simulink model "A1_VSC_3phase"  (R2024b)
settings: Solver=ode1  StartTime=0.0  StopTime=tsim  FixedStep=tsamp  RelTol=1e-3
values from neighbouring files (symbols this model uses):
  conv = 4    [A1_VSC_3phase.m]
  fsw = 35e3    (= 35000)    [A1_VSC_3phase.m]
  kd = sqrt(2/3)    [A1_VSC_3phase.m]
  Ki = 2*pi*fsw*req/10    (= 659.734457254)    [A1_VSC_3phase.m]
  ko = sqrt(1/3)    [A1_VSC_3phase.m]
  Kp = 2*pi*fsw*Lg/10    (= 43.9822971503)    [A1_VSC_3phase.m]
  Lg = 2e-3    (= 0.002)    [A1_VSC_3phase.m]
  P1 = -5e3    (= -5000)    [A1_VSC_3phase.m]
  P2 = 1e3    (= 1000)    [A1_VSC_3phase.m]
  P3 = 5e3    (= 5000)    [A1_VSC_3phase.m]
  P4 = -5e3    (= -5000)    [A1_VSC_3phase.m]
  rg = 10e-3    (= 0.01)    [A1_VSC_3phase.m]
  tsamp = 1/(samples_per_switching*fsw)    (= 2.85714285714e-07)    [A1_VSC_3phase.m]
  Vdc = 800    [A1_VSC_3phase.m]
  Vg1 = 428    [A1_VSC_3phase.m]
  Vg2 = 438    [A1_VSC_3phase.m]
  Vg3 = 438    [A1_VSC_3phase.m]
  Vg4 = 438    [A1_VSC_3phase.m]
libraries: spsMosfetLib x6, spsVoltageMeasurementLib x4, spsControlledVoltageSourceLib x3, spsCurrentMeasurementLib x3, spsSeriesRLCBranchLib x3, slpidlib x2, spsStairGeneratorLib x2, spsDCVoltageSourceLib x1, simulink x1, spsGroundLib x1, spsPLL3phLib x1, spspowerguiLib x1
settings Model: Creator=Admin  LastModifiedBy=admin
settings RTWCC: GPUComputeCapability=3.5

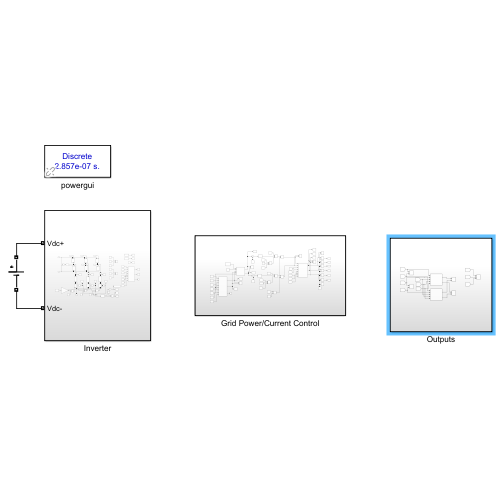
[thumbnail: Simulink's stored preview of the top-level diagram]
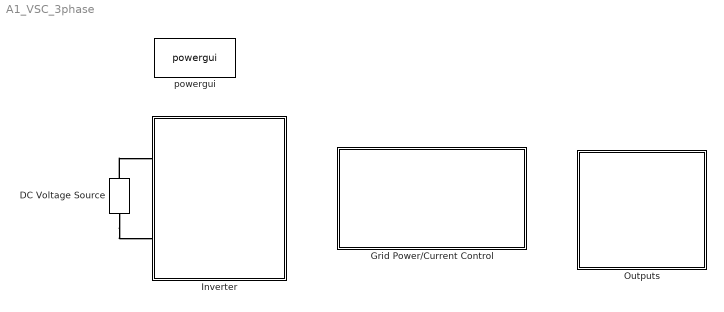
== system A1_VSC_3phase ==
  DC Voltage Source : spsDCVoltageSourceLib/DC Voltage Source  Amplitude=Vdc  Measurements=None
  Grid Power/Current Control : Subsystem
  Inverter : Subsystem
  Outputs : Subsystem
  powergui : spspowerguiLib/powergui  Priority=1  SimulationMode=Discrete  SampleTime=tsamp  frequency=60  Iterations=50  frequencyindice=0  Pbase=100e6  ErrMax=1e-4  UnitsV=kV  UnitsW=MW  buscounter=0  FunctionMessages=off  echomessages=off  EnableUseOfTLC=off  CurrentSourceSwitches=off  DisableSnubberDevices=off  DisableRonSwitches=off  DisableVfSwitches=off  DisplayEquations=off  AutomaticDiscreteSolvers=off  SolverType=Tustin/Backward Euler (TBE)  Interpol=off  ExternalGateDelay=off  methode=off  Ts=100  x0status=blocks  SPID=on  SwTol=0  HookPort=off  NonlinearTolerance=1e-4  nMaxIteration=100  ContinueOnMaxIteration=off  RestoreLinks=warning  ResistiveCurrentMeasurement=off  Frange=[0:2:500]  Ylog=off  Xlog=on  ShowGrid=off  save=off  variable=ZData  structure=0  ZoomFFT=off  StartTime=0.0  cycles=1  DisplayStyle=1  fundamental=60  FreqAxis=off  MaxFrequency=1000  frequencyindicesteady=1  RmsSteady=1  display=off
  connections:
  DC Voltage Source/LConn1 -- Inverter/LConn2
  DC Voltage Source/RConn1 -- Inverter/LConn1

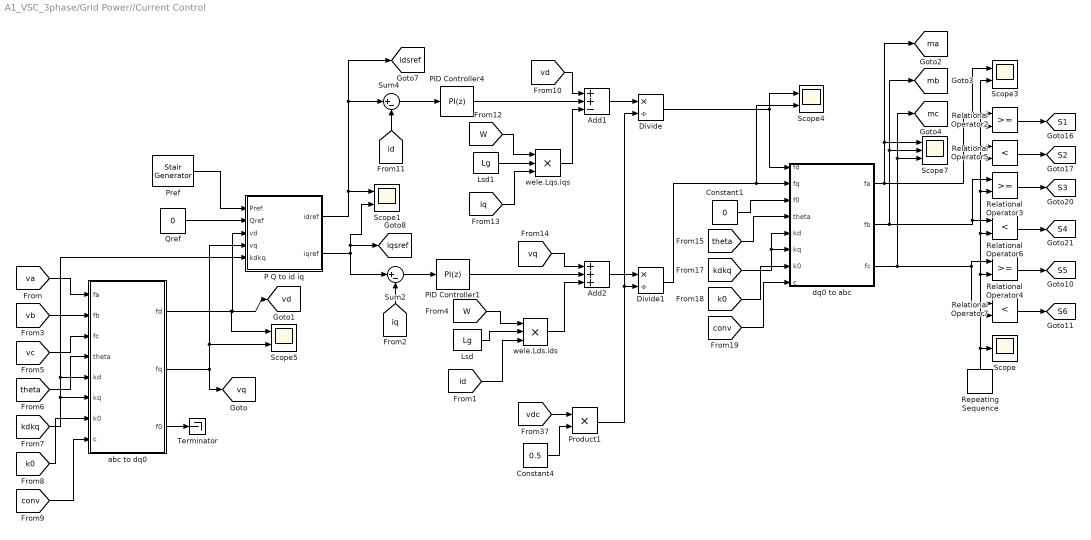
== system A1_VSC_3phase/Grid Power//Current Control ==
  Add1 : Sum  Inputs=++-
  Add2 : Sum  Inputs=+++
  Constant1 : Constant  Value=0
  Constant4 : Constant  Value=0.5
  Divide : Product  Inputs=*/
  Divide1 : Product  Inputs=*/
  Lsd : Constant  Value=Lg
  Lsd1 : Constant  Value=Lg
  P Q to id iq : MATLAB Function  TreatAsAtomicUnit=on
  PID Controller1 : slpidlib/PID Controller  Controller=PI  Form=Parallel  TimeDomain=Discrete-time  UseExternalTs=off  SampleTime=tsamp  IntegratorMethod=Forward Euler  FilterMethod=Forward Euler  ControllerParametersSource=internal  P=Kp  I=Ki  UseKiTs=off  D=0  UseExternalDerivativeSource=off  N=100  UseFilter=on  TunerSelectOption=Transfer Function Based (PID Tuner App)  InitialConditionSource=internal  InitialConditionForIntegrator=0  InitialConditionForFilter=0  DifferentiatorICPrevScaledInput=0  ExternalReset=none  TrackingMode=off  Kt=1  LimitOutput=off  SatLimitsSource=internal  UpperSaturationLimit=inf  LowerSaturationLimit=-inf  LinearizeAsGain=on  AntiWindupMode=none  Kb=1  LimitIntegrator=off  UpperIntegratorSaturationLimit=inf  LowerIntegratorSaturationLimit=-inf  POutMin=[]  POutMax=[]  IOutMin=[]  IOutMax=[]  DOutMin=[]  DOutMax=[]  NOutMin=[]  NOutMax=[]  SumOutMin=[]  SumOutMax=[]  SaturationOutMin=[]  SaturationOutMax=[]  PParamMin=[]  PParamMax=[]  IParamMin=[]  IParamMax=[]  DParamMin=[]  DParamMax=[]  NParamMin=[]  NParamMax=[]  KbParamMin=[]  KbParamMax=[]  KtParamMin=[]  KtParamMax=[]  KbOutMin=[]  KbOutMax=[]  KtOutMin=[]  KtOutMax=[]  IntegratorOutMin=[]  IntegratorOutMax=[]  FilterOutMin=[]  FilterOutMax=[]  SumI1OutMin=[]  SumI1OutMax=[]  SumI2OutMin=[]  SumI2OutMax=[]  SumI3OutMin=[]  SumI3OutMax=[]  SumI4OutMin=[]  SumI4OutMax=[]  SumDOutMin=[]  SumDOutMax=[]  DifferentiatorOutMin=[]  DifferentiatorOutMax=[]  FilterDiffOutCoefMin=[]  FilterDiffOutCoefMax=[]  ReciprocalOutMin=[]  ReciprocalOutMax=[]  SumDenOutMin=[]  SumDenOutMax=[]  SumNumOutMin=[]  SumNumOutMax=[]  DivideOutMin=[]  DivideOutMax=[]  UdiffTsProdOutMin=[]  UdiffTsProdOutMax=[]  NTsProdOutMin=[]  NTsProdOutMax=[]  UintegralTsProdOutMin=[]  UintegralTsProdOutMax=[]  UngainTsProdOutMin=[]  UngainTsProdOutMax=[]  ClampingZeroOutDataTypeStr=Inherit: Inherit via back propagation  ClampingZeroOutMin=[]  ClampingZeroOutMax=[]  FilterDenConstantOutDataTypeStr=Inherit: Inherit via back propagation  FilterDenConstantOutMin=[]  FilterDenConstantOutMax=[]  PCopyOutDataTypeStr=Inherit: Inherit via back propagation  PCopyOutMin=[]  PCopyOutMax=[]  NCopyOutDataTypeStr=Inherit: Inherit via back propagation  NCopyOutMin=[]  NCopyOutMax=[]  IntegratorContinuousStateAttributes=''  IntegratorStateMustResolveToSignalObject=off  IntegratorRTWStateStorageClass=Auto  FilterContinuousStateAttributes=''  FilterStateMustResolveToSignalObject=off  FilterRTWStateStorageClass=Auto  ParallelPVariant=InternalParameters  IdealPVariant=Disabled  IVariant=InternalParameters  DVariant=Disabled  IntegratorVariant=Discrete  SatVariant=Disabled  AWVariant=Passthrough  PCopyVariant=Disabled  TRVariant=Disabled  FdbkBlocksVariant=Forward  IdealPFdbkVariant=Disabled  SatFdbkVariant=Disabled  DerivativeFilterVariant=Disabled  NVariant=Disabled  NCopyVariant=Disabled_SignalSpec  FilterICVariant=Disabled  IntegratorICVariant=InternalICs  ExternalResetVariant=Disabled  TRSumVariant=Passthrough  SumFdbkVariant=Disabled  SumVariant=Sum_PI  TsampFilterVariant=InternalTs  TsampNgainVariant=Passthrough  TsampIntegralVariant=Disabled_SignalSpec  ExternalSaturationOutDataTypeStr=Inherit: Same as second input  DerivativeSourceVariant=Disabled  PreIntVariant=InternalPreInt
  PID Controller4 : slpidlib/PID Controller  Controller=PI  Form=Parallel  TimeDomain=Discrete-time  UseExternalTs=off  SampleTime=tsamp  IntegratorMethod=Forward Euler  FilterMethod=Forward Euler  ControllerParametersSource=internal  P=Kp  I=Ki  UseKiTs=off  D=0  UseExternalDerivativeSource=off  N=100  UseFilter=on  TunerSelectOption=Transfer Function Based (PID Tuner App)  InitialConditionSource=internal  InitialConditionForIntegrator=0  InitialConditionForFilter=0  DifferentiatorICPrevScaledInput=0  ExternalReset=none  TrackingMode=off  Kt=1  LimitOutput=off  SatLimitsSource=internal  UpperSaturationLimit=inf  LowerSaturationLimit=-inf  LinearizeAsGain=on  AntiWindupMode=none  Kb=1  LimitIntegrator=off  UpperIntegratorSaturationLimit=inf  LowerIntegratorSaturationLimit=-inf  POutMin=[]  POutMax=[]  IOutMin=[]  IOutMax=[]  DOutMin=[]  DOutMax=[]  NOutMin=[]  NOutMax=[]  SumOutMin=[]  SumOutMax=[]  SaturationOutMin=[]  SaturationOutMax=[]  PParamMin=[]  PParamMax=[]  IParamMin=[]  IParamMax=[]  DParamMin=[]  DParamMax=[]  NParamMin=[]  NParamMax=[]  KbParamMin=[]  KbParamMax=[]  KtParamMin=[]  KtParamMax=[]  KbOutMin=[]  KbOutMax=[]  KtOutMin=[]  KtOutMax=[]  IntegratorOutMin=[]  IntegratorOutMax=[]  FilterOutMin=[]  FilterOutMax=[]  SumI1OutMin=[]  SumI1OutMax=[]  SumI2OutMin=[]  SumI2OutMax=[]  SumI3OutMin=[]  SumI3OutMax=[]  SumI4OutMin=[]  SumI4OutMax=[]  SumDOutMin=[]  SumDOutMax=[]  DifferentiatorOutMin=[]  DifferentiatorOutMax=[]  FilterDiffOutCoefMin=[]  FilterDiffOutCoefMax=[]  ReciprocalOutMin=[]  ReciprocalOutMax=[]  SumDenOutMin=[]  SumDenOutMax=[]  SumNumOutMin=[]  SumNumOutMax=[]  DivideOutMin=[]  DivideOutMax=[]  UdiffTsProdOutMin=[]  UdiffTsProdOutMax=[]  NTsProdOutMin=[]  NTsProdOutMax=[]  UintegralTsProdOutMin=[]  UintegralTsProdOutMax=[]  UngainTsProdOutMin=[]  UngainTsProdOutMax=[]  ClampingZeroOutDataTypeStr=Inherit: Inherit via back propagation  ClampingZeroOutMin=[]  ClampingZeroOutMax=[]  FilterDenConstantOutDataTypeStr=Inherit: Inherit via back propagation  FilterDenConstantOutMin=[]  FilterDenConstantOutMax=[]  PCopyOutDataTypeStr=Inherit: Inherit via back propagation  PCopyOutMin=[]  PCopyOutMax=[]  NCopyOutDataTypeStr=Inherit: Inherit via back propagation  NCopyOutMin=[]  NCopyOutMax=[]  IntegratorContinuousStateAttributes=''  IntegratorStateMustResolveToSignalObject=off  IntegratorRTWStateStorageClass=Auto  FilterContinuousStateAttributes=''  FilterStateMustResolveToSignalObject=off  FilterRTWStateStorageClass=Auto  ParallelPVariant=InternalParameters  IdealPVariant=Disabled  IVariant=InternalParameters  DVariant=Disabled  IntegratorVariant=Discrete  SatVariant=Disabled  AWVariant=Passthrough  PCopyVariant=Disabled  TRVariant=Disabled  FdbkBlocksVariant=Forward  IdealPFdbkVariant=Disabled  SatFdbkVariant=Disabled  DerivativeFilterVariant=Disabled  NVariant=Disabled  NCopyVariant=Disabled_SignalSpec  FilterICVariant=Disabled  IntegratorICVariant=InternalICs  ExternalResetVariant=Disabled  TRSumVariant=Passthrough  SumFdbkVariant=Disabled  SumVariant=Sum_PI  TsampFilterVariant=InternalTs  TsampNgainVariant=Passthrough  TsampIntegralVariant=Disabled_SignalSpec  ExternalSaturationOutDataTypeStr=Inherit: Same as second input  DerivativeSourceVariant=Disabled  PreIntVariant=InternalPreInt
  Pref : spsStairGeneratorLib/Stair Generator  t=[0 0.25 0.5 0.75]  e=[P1 P2 P3 P4]  Ts=0
  Product1 : Product
  Qref : Constant  Value=0
  Relational Operator2 : RelationalOperator  OutDataTypeStr=boolean  RndMeth=Simplest  InputSameDT=off
  Relational Operator3 : RelationalOperator  OutDataTypeStr=boolean  RndMeth=Simplest  InputSameDT=off
  Relational Operator4 : RelationalOperator  OutDataTypeStr=boolean  RndMeth=Simplest  InputSameDT=off
  Relational Operator5 : RelationalOperator  Operator=<  OutDataTypeStr=boolean  RndMeth=Simplest  InputSameDT=off
  Relational Operator6 : RelationalOperator  Operator=<  OutDataTypeStr=boolean  RndMeth=Simplest  InputSameDT=off
  Relational Operator7 : RelationalOperator  Operator=<  OutDataTypeStr=boolean  RndMeth=Simplest  InputSameDT=off
  Repeating Sequence : simulink/Sources/Repeating Sequence  rep_seq_t=[0 1/(4*fsw) 1/(2*fsw) 3/(4*fsw) 1/(fsw)]  rep_seq_y=[0 0.5 1 0.5 0]
  Scope : Scope
  Scope{1,3..5} (4 alike) : Scope  NumInputPorts=2
  Scope7 : Scope  NumInputPorts=3
  Sum2 : Sum  Inputs=|+-
  Sum4 : Sum  Inputs=|+-
  Terminator : Terminator
  abc to dq0 : MATLAB Function  TreatAsAtomicUnit=on
  dq0 to abc : MATLAB Function  TreatAsAtomicUnit=on
  wele.Lds.ids : Product  Inputs=3
  wele.Lqs.iqs : Product  Inputs=3
  tag scope: S1=global, S2=global, S3=global, S4=global, S5=global, S6=global, idsref=global, iqsref=global, ma=global, mb=global, mc=global, vd=global, vq=global
  wires:
  Relational Operator2/1 -> [S1]
  [W] -> wele.Lqs.iqs/1
  dq0 to abc/1(fa) -> [ma], Scope7/1, Relational Operator2/1, Scope3/1, Relational Operator5/1
  Product1/1 -> Divide/2, Divide1/2
  [theta] -> dq0 to abc/4(theta)
  [kdkq] -> dq0 to abc/6(kq), dq0 to abc/5(kd)
  [W] -> wele.Lds.ids/1
  Constant1/1 -> dq0 to abc/3(f0)
  Sum2/1 -> PID Controller1/1
  Lsd1/1 -> wele.Lqs.iqs/2
  Sum4/1 -> PID Controller4/1
  [vdc] -> Product1/1
  [iq] -> Sum2/2
  Relational Operator4/1 -> [S5]
  Relational Operator5/1 -> [S2]
  Constant4/1 -> Product1/2
  Lsd/1 -> wele.Lds.ids/2
  Relational Operator3/1 -> [S3]
  [iq] -> wele.Lqs.iqs/3
  dq0 to abc/3(fc) -> [mc], Scope7/3, Relational Operator4/1, Relational Operator7/1
  [id] -> wele.Lds.ids/3
  dq0 to abc/2(fb) -> [mb], Scope7/2, Relational Operator6/1, Relational Operator3/1
  [id] -> Sum4/2
  Relational Operator7/1 -> [S6]
  [conv] -> dq0 to abc/8(c)
  Repeating Sequence/1 -> Scope/1, Relational Operator2/2, Scope3/2, Relational Operator5/2, Relational Operator3/2, Relational Operator6/2, Relational Operator4/2, Relational Operator7/2
  Divide/1 -> dq0 to abc/1(fd), Scope4/1
  Relational Operator6/1 -> [S4]
  Divide1/1 -> Scope4/2, dq0 to abc/2(fq)
  [k0] -> dq0 to abc/7(k0)
  P Q to id iq/2(iqref) -> Sum2/1, Scope1/2, [iqsref]
  P Q to id iq/1(idref) -> Scope1/1, Sum4/1, [idsref]
  Pref/1 -> P Q to id iq/1(Pref)
  Qref/1 -> P Q to id iq/2(Qref)
  [va] -> abc to dq0/1(fa)
  [vc] -> abc to dq0/3(fc)
  [vb] -> abc to dq0/2(fb)
  [theta] -> abc to dq0/4(theta)
  [kdkq] -> abc to dq0/6(kq), P Q to id iq/5(kdkq), abc to dq0/5(kd)
  [k0] -> abc to dq0/7(k0)
  [conv] -> abc to dq0/8(c)
  abc to dq0/2(fq) -> Scope5/2, P Q to id iq/4(vq), [vq]
  abc to dq0/3(f0) -> Terminator/1
  abc to dq0/1(fd) -> [vd], P Q to id iq/3(vd), Scope5/1
  PID Controller4/1 -> Add1/2
  PID Controller1/1 -> Add2/2
  [vd] -> Add1/1
  [vq] -> Add2/1
  wele.Lds.ids/1 -> Add2/3
  wele.Lqs.iqs/1 -> Add1/3
  Add1/1 -> Divide/1
  Add2/1 -> Divide1/1

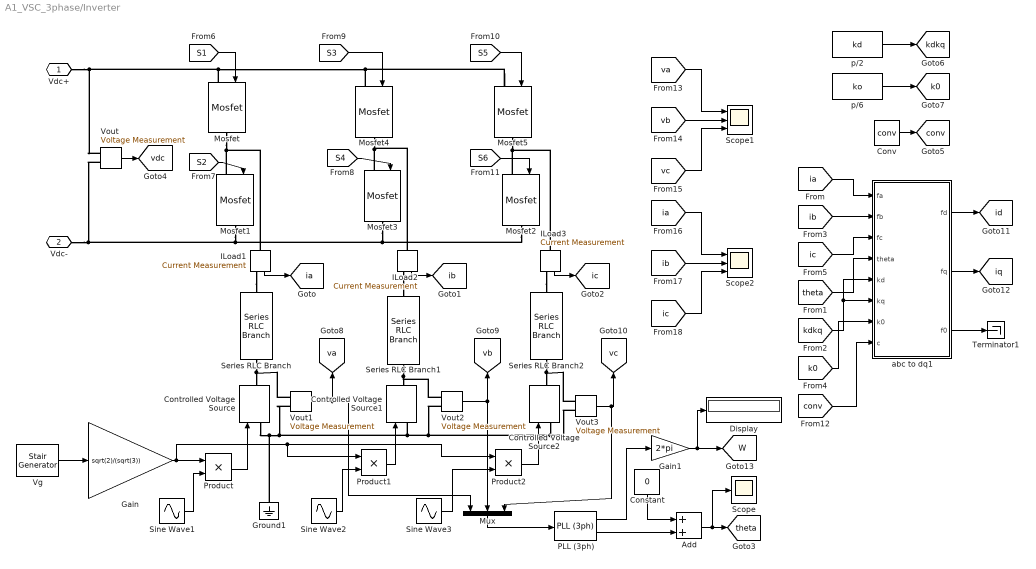
== system A1_VSC_3phase/Inverter ==
  Add : Sum
  Constant : Constant  Value=0
  Controlled Voltage Source : spsControlledVoltageSourceLib/Controlled Voltage Source  Initialize=on  Source_Type=AC  Amplitude=0  Phase=0  Frequency=50  Measurements=None
  Controlled Voltage Source1 : spsControlledVoltageSourceLib/Controlled Voltage Source  Initialize=on  Source_Type=AC  Amplitude=0  Phase=0  Frequency=50  Measurements=None
  Controlled Voltage Source2 : spsControlledVoltageSourceLib/Controlled Voltage Source  Initialize=on  Source_Type=AC  Amplitude=0  Phase=0  Frequency=50  Measurements=None
  Conv : Constant  Value=conv
  Display : Display
  Gain : Gain  Gain=sqrt(2)/(sqrt(3))
  Gain1 : Gain  Gain=2*pi
  Ground1 : spsGroundLib/Ground  LConnTagsString=a
  ILoad1 : spsCurrentMeasurementLib/Current Measurement  PhasorSimulation=off  OutputType=Complex  PSBequivalent=0
  ILoad2 : spsCurrentMeasurementLib/Current Measurement  PhasorSimulation=off  OutputType=Complex  PSBequivalent=0
  ILoad3 : spsCurrentMeasurementLib/Current Measurement  PhasorSimulation=off  OutputType=Complex  PSBequivalent=0
  Mosfet{,1..5} (6 alike) : spsMosfetLib/Mosfet  Ron=rdson  Lon=0  Rd=0.01  Vfd=0  IC=0  Rs=1e5  Cs=inf  Measurements=off
  Mux : Mux  Inputs=3
  PLL (3ph) : spsPLL3phLib/PLL (3ph)  Fmin=50  Par_Init=[0, 50]  ParK=[180, 3200, 1]  TcD=1e-4  MaxRateChangeFreq=12  FilterCutOffFreq=25  Ts=0  AGC=on
  Product : Product
  Product1 : Product
  Product2 : Product
  Scope : Scope
  Scope1 : Scope  NumInputPorts=3
  Scope2 : Scope  NumInputPorts=3
  Series RLC Branch : spsSeriesRLCBranchLib/Series RLC Branch  LConnTagsString=__new0  RConnTagsString=__new0  BranchType=RL  Resistance=rg  Inductance=Lg  SetiL0=off  InitialCurrent=0  Capacitance=1e-6  Setx0=off  InitialVoltage=0  Measurements=None
  Series RLC Branch1 : spsSeriesRLCBranchLib/Series RLC Branch  LConnTagsString=__new0  RConnTagsString=__new0  BranchType=RL  Resistance=rg  Inductance=Lg  SetiL0=off  InitialCurrent=0  Capacitance=1e-6  Setx0=off  InitialVoltage=0  Measurements=None
  Series RLC Branch2 : spsSeriesRLCBranchLib/Series RLC Branch  LConnTagsString=__new0  RConnTagsString=__new0  BranchType=RL  Resistance=rg  Inductance=Lg  SetiL0=off  InitialCurrent=0  Capacitance=1e-6  Setx0=off  InitialVoltage=0  Measurements=None
  Sine Wave1 : Sin  Frequency=100*pi
  Sine Wave2 : Sin  Frequency=100*pi  Phase=-2*pi/3
  Sine Wave3 : Sin  Frequency=100*pi  Phase=2*pi/3
  Terminator1 : Terminator
  Vg : spsStairGeneratorLib/Stair Generator  t=[0 0.25 0.5 0.75]  e=[Vg1 Vg2 Vg3 Vg4]  Ts=0
  Vout{,1..3} (4 alike) : spsVoltageMeasurementLib/Voltage Measurement  PhasorSimulation=off  OutputType=Complex  PSBequivalent=0
  abc to dq1 : MATLAB Function  TreatAsAtomicUnit=on
  p/2 : Constant  Value=kd
  p/6 : Constant  Value=ko
  Vdc+ : PMIOPort  Side=Left
  Vdc- : PMIOPort  Port=2  Side=Left
  tag scope: W=global, conv=global, ia=global, ib=global, ic=global, id=global, iq=global, k0=global, kdkq=global, theta=global, va=global, vb=global, vc=global, vdc=global
  wires:
  Vout/1 -> [vdc]
  Vg/1 -> Gain/1
  ILoad1/1 -> [ia]
  ILoad2/1 -> [ib]
  ILoad3/1 -> [ic]
  Product/1 -> Controlled Voltage Source/1
  PLL (3ph)/2 -> Add/2
  Mux/1 -> PLL (3ph)/1
  PLL (3ph)/1 -> Gain1/1
  Vout1/1 -> Mux/1, [va]
  Vout2/1 -> [vb], Mux/2
  Vout3/1 -> Mux/3, [vc]
  p/2/1 -> [kdkq]
  p/6/1 -> [k0]
  Conv/1 -> [conv]
  Add/1 -> Scope/1, [theta]
  Constant/1 -> Add/1
  [theta] -> abc to dq1/4(theta)
  [ia] -> abc to dq1/1(fa)
  [ic] -> abc to dq1/3(fc)
  [conv] -> abc to dq1/8(c)
  [kdkq] -> abc to dq1/6(kq), abc to dq1/5(kd)
  [ib] -> abc to dq1/2(fb)
  [k0] -> abc to dq1/7(k0)
  abc to dq1/2(fq) -> [iq]
  abc to dq1/3(f0) -> Terminator1/1
  abc to dq1/1(fd) -> [id]
  Gain1/1 -> Display/1, [W]
  [va] -> Scope1/1
  [vb] -> Scope1/2
  [vc] -> Scope1/3
  [ic] -> Scope2/3
  [ib] -> Scope2/2
  [ia] -> Scope2/1
  [S1] -> Mosfet/1
  [S2] -> Mosfet1/1
  [S3] -> Mosfet4/1
  [S4] -> Mosfet3/1
  [S5] -> Mosfet5/1
  [S6] -> Mosfet2/1
  Product1/1 -> Controlled Voltage Source1/1
  Product2/1 -> Controlled Voltage Source2/1
  Gain/1 -> Product2/1, Product1/1, Product/1
  Sine Wave1/1 -> Product/2
  Sine Wave2/1 -> Product1/2
  Sine Wave3/1 -> Product2/2
  connections:
  ILoad1/LConn1 -- Mosfet1/LConn1 -- Mosfet/RConn1
  Vout/LConn1 -- Mosfet5/LConn1 -- Mosfet4/LConn1 -- Mosfet/LConn1 -- Vdc+/RConn1
  ILoad3/LConn1 -- Mosfet2/LConn1 -- Mosfet5/RConn1
  ILoad2/LConn1 -- Mosfet4/RConn1 -- Mosfet3/LConn1
  Mosfet2/RConn1 -- Mosfet3/RConn1 -- Mosfet1/RConn1 -- Vdc-/RConn1 -- Vout/LConn2
  Controlled Voltage Source/LConn1 -- Ground1/LConn1 -- Vout1/LConn2 -- Vout3/LConn2 -- Controlled Voltage Source2/LConn1 -- Vout2/LConn2 -- Controlled Voltage Source1/LConn1
  Series RLC Branch/RConn1 -- Vout1/LConn1 -- Controlled Voltage Source/RConn1
  Series RLC Branch1/RConn1 -- Controlled Voltage Source1/RConn1 -- Vout2/LConn1
  ILoad3/RConn1 -- Series RLC Branch2/LConn1
  ILoad1/RConn1 -- Series RLC Branch/LConn1
  ILoad2/RConn1 -- Series RLC Branch1/LConn1
  Series RLC Branch2/RConn1 -- Vout3/LConn1 -- Controlled Voltage Source2/RConn1

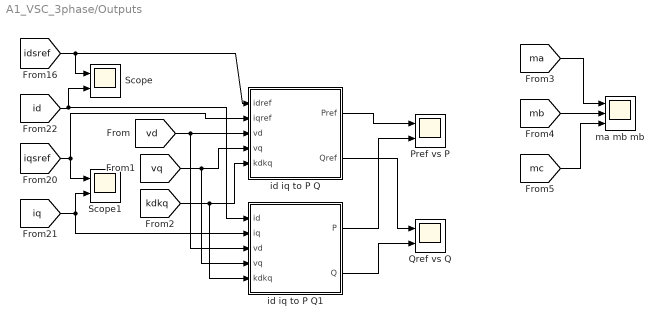
== system A1_VSC_3phase/Outputs ==
  Pref vs P : Scope  NumInputPorts=2
  Qref vs Q : Scope  NumInputPorts=2
  Scope : Scope  NumInputPorts=2
  Scope1 : Scope  NumInputPorts=2
  id iq to P Q : MATLAB Function  TreatAsAtomicUnit=on
  id iq to P Q1 : MATLAB Function  TreatAsAtomicUnit=on
  ma mb mb : Scope  NumInputPorts=3
  wires:
  [idsref] -> Scope/1, id iq to P Q/1(idref)
  [id] -> id iq to P Q1/1(id), Scope/2
  [iqsref] -> Scope1/1, id iq to P Q/2(iqref)
  [iq] -> Scope1/2, id iq to P Q1/2(iq)
  [vd] -> id iq to P Q1/3(vd), id iq to P Q/3(vd)
  [vq] -> id iq to P Q1/4(vq), id iq to P Q/4(vq)
  [kdkq] -> id iq to P Q1/5(kdkq), id iq to P Q/5(kdkq)
  id iq to P Q/1(Pref) -> Pref vs P/1
  id iq to P Q1/1(P) -> Pref vs P/2
  id iq to P Q/2(Qref) -> Qref vs Q/1
  id iq to P Q1/2(Q) -> Qref vs Q/2
  [ma] -> ma mb mb/1
  [mb] -> ma mb mb/2
  [mc] -> ma mb mb/3

== matlab function A1_VSC_3phase/Outputs/id iq to P Q ==
  data: idref input; Pref output; iqref input; vd input; vq input; Qref output; kdkq input
function [Pref, Qref] = fcn(idref, iqref, vd, vq, kdkq)

Pref=(2/(3*kdkq^2))*(vd*idref+vq*iqref);
Qref=(2/(3*kdkq^2))*(vq*idref-vd*iqref);

== matlab function A1_VSC_3phase/Outputs/id iq to P Q1 ==
  data: id input; P output; iq input; vd input; vq input; Q output; kdkq input
function [P, Q] = fcn(id, iq, vd, vq, kdkq)

P=(2/(3*kdkq^2))*(vd*id+vq*iq);
Q=(2/(3*kdkq^2))*(vq*id-vd*iq);

== matlab function A1_VSC_3phase/Grid Power//Current Control/P Q to id iq ==
  data: Pref input; idref output; Qref input; vd input; vq input; iqref output; kdkq input
function [idref, iqref] = fcn(Pref, Qref, vd, vq, kdkq)

idref=1.5*kdkq^2*(vd*Pref+vq*Qref)/(vd^2+vq^2);
iqref=1.5*kdkq^2*(vq*Pref-vd*Qref)/(vd^2+vq^2);

== matlab function A1_VSC_3phase/Grid Power//Current Control/abc to dq0 ==
  data: fa input; fd output; fb input; fc input; theta input; fq output; f0 output; kd input; kq input; k0 input; c input
function [fd, fq, f0] = fcn(fa, fb, fc, theta, kd, kq, k0, c)

if c==1
    psi = 0;
    sigma = 1;
elseif c==2
    psi = pi/2;
    sigma = 1;
elseif c==3
    psi = 0;
    sigma = -1;
else
    psi = -pi/2;
    sigma = -1;
end

fd = kd*cos(theta+psi)*fa + kd*cos(theta+psi-2*pi/3)*fb + kd*cos(theta+psi+2*pi/3)*fc;
fq = sigma*kq*sin(theta+psi)*fa + sigma*kq*sin(theta+psi-2*pi/3)*fb + sigma*kq*sin(theta+psi+2*pi/3)*fc;
f0 = k0*fa + k0*fb + k0*fc;

== matlab function A1_VSC_3phase/Inverter/abc to dq1 ==
  data: fa input; fd output; fb input; fc input; theta input; fq output; f0 output; kd input; kq input; k0 input; c input
function [fd, fq, f0] = fcn(fa, fb, fc, theta, kd, kq, k0, c)

if c==1
    psi = 0;
    sigma = 1;
elseif c==2
    psi = pi/2;
    sigma = 1;
elseif c==3
    psi = 0;
    sigma = -1;
else
    psi = -pi/2;
    sigma = -1;
end

fd = kd*cos(theta+psi)*fa + kd*cos(theta+psi-2*pi/3)*fb + kd*cos(theta+psi+2*pi/3)*fc;
fq = sigma*kq*sin(theta+psi)*fa + sigma*kq*sin(theta+psi-2*pi/3)*fb + sigma*kq*sin(theta+psi+2*pi/3)*fc;
f0 = k0*fa + k0*fb + k0*fc;

== matlab function A1_VSC_3phase/Grid Power//Current Control/dq0 to abc ==
  data: fd input; fa output; fq input; f0 input; theta input; fb output; fc output; kd input; kq input; k0 input; c input
function [fa, fb, fc] = fcn(fd, fq, f0, theta, kd, kq, k0, c)

if c==1
    psi = 0;
    sigma = 1;
elseif c==2
    psi = pi/2;
    sigma = 1;
elseif c==3
    psi = 0;
    sigma = -1;
else
    psi = -pi/2;
    sigma = -1;
end

k1 = 2/(3*kd);
k2 = 2/(3*kq);
k3 = 1/(3*k0);
fa = k1*cos(theta+psi)*fd + sigma*k2*sin(theta+psi)*fq + k3*f0;
fb = k1*cos(theta+psi-2*pi/3)*fd + sigma*k2*sin(theta+psi-2*pi/3)*fq + k3*f0;
fc = k1*cos(theta+psi+2*pi/3)*fd + sigma*k2*sin(theta+psi+2*pi/3)*fq + k3*f0;
